simulink library "aerolib6dofsys"  (Simulink 5.0)
undefined symbols (not defined in the file or in its folder): e0_0, e1_0, e2_0, e3_0, eul_0, inertia, k_quat, mass_0, mass_e, mass_f
libraries: aerolibtransform2 x4, simulink x3, aerolibutil x1, aerolibbdyn x1
settings Model: Creator=sgage  LastModifiedBy=sgage  ExtModeAutoUpdateStatusClock=off  TargetHWChar=2  TargetHWWordLengths=8,16,32,32

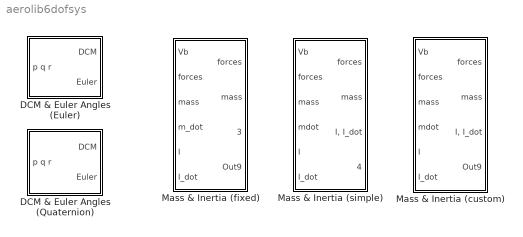
== system aerolib6dofsys ==
  DCM & Euler Angles (Euler) : Subsystem
      mask Type: DCM & Euler Angles (Euler)
  DCM & Euler Angles (Quaternion) : Subsystem
      mask Type: DCM & Euler Angles (Quaternion)
  Mass & Inertia (custom) : Subsystem
      mask Type: Mass & Inertia (custom)
  Mass & Inertia (fixed) : Subsystem
      mask Type: Mass & Inertia (fixed)
  Mass & Inertia (simple) : Subsystem
      mask Type: Mass & Inertia (simple)

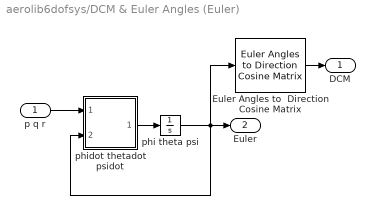
== system aerolib6dofsys/DCM & Euler Angles (Euler) ==
  "p q r " : Inport
  Euler Angles to  Direction Cosine Matrix : aerolibtransform2/Euler Angles to  Direction Cosine Matrix
  phi theta psi : Integrator  InitialCondition=eul_0
  phidot thetadot psidot : Subsystem
  DCM : Outport
  Euler : Outport  Port=2
  wires:
  Euler Angles to  Direction Cosine Matrix/1 -> DCM/1
  "p q r "/1 -> phidot thetadot psidot/1(p q r)
  phidot thetadot psidot/1(phidot thetadot psi) -> phi theta psi/1
  phi theta psi/1 -> Euler/1, phidot thetadot psidot/2(phi theta psi), Euler Angles to  Direction Cosine Matrix/1

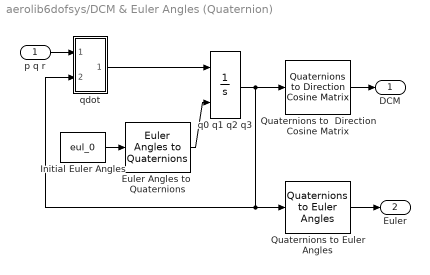
== system aerolib6dofsys/DCM & Euler Angles (Quaternion) ==
  p q r : Inport
  Euler Angles to  Quaternions : aerolibtransform2/Euler Angles to Quaternions
  Initial Euler Angles : Constant  Value=eul_0
  Quaternions to  Direction Cosine Matrix : aerolibtransform2/Quaternions to  Direction Cosine Matrix
  Quaternions to Euler Angles : aerolibtransform2/Quaternions to Euler Angles
  q0 q1 q2 q3 : Integrator  InitialConditionSource=external  InitialCondition=[e0_0 e1_0 e2_0 e3_0]
  qdot : Subsystem
  DCM : Outport
  Euler : Outport  Port=2
  wires:
  qdot/1(qdot) -> q0 q1 q2 q3/1
  q0 q1 q2 q3/1 -> qdot/2(q0 q1 q2 q3), Quaternions to Euler Angles/1, Quaternions to  Direction Cosine Matrix/1
  Euler Angles to  Quaternions/1 -> q0 q1 q2 q3/2
  Initial Euler Angles/1 -> Euler Angles to  Quaternions/1
  p q r/1 -> qdot/1(p q r)
  Quaternions to  Direction Cosine Matrix/1 -> DCM/1
  Quaternions to Euler Angles/1 -> Euler/1

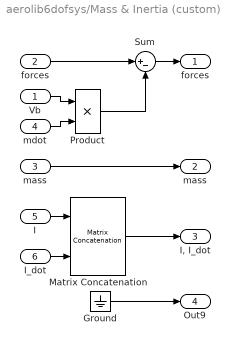
== system aerolib6dofsys/Mass & Inertia (custom) ==
  Vb : Inport
  forces : Inport  Port=2
  "mass " : Inport  Port=3
  mdot : Inport  Port=4
  I : Inport  Port=5
  I_dot : Inport  Port=6
  Ground : Ground
  Matrix Concatenation : simulink/Math Operations/Matrix Concatenation  numInports=2  catMethod=Vertical
  Product : Product  SaturateOnIntegerOverflow=on
  Sum : Sum  Inputs=|+-  SaturateOnIntegerOverflow=on
  "forces " : Outport
  mass : Outport  Port=2
  "I, I_dot " : Outport  Port=3
  Out9 : Outport  Port=4
  wires:
  Ground/1 -> Out9/1
  I/1 -> Matrix Concatenation/1
  "mass "/1 -> mass/1
  Matrix Concatenation/1 -> "I, I_dot "/1
  I_dot/1 -> Matrix Concatenation/2
  mdot/1 -> Product/2
  forces/1 -> Sum/1
  Vb/1 -> Product/1
  Sum/1 -> "forces "/1
  Product/1 -> Sum/2

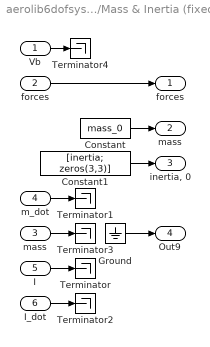
== system aerolib6dofsys/Mass & Inertia (fixed) ==
  Vb : Inport
  forces : Inport  Port=2
  "mass " : Inport  Port=3
  m_dot : Inport  Port=4  ShowAdditionalParam=on  DataType=double
  I : Inport  Port=5  ShowAdditionalParam=on  DataType=double
  I_dot : Inport  Port=6  ShowAdditionalParam=on  DataType=double
  Constant : Constant  Value=mass_0  ShowAdditionalParam=on
  Constant1 : Constant  Value=[inertia; zeros(3,3)]  ShowAdditionalParam=on
  Ground : Ground
  Terminator{,1..4} (5 alike) : Terminator
  "forces " : Outport
  mass : Outport  Port=2
  "inertia, 0" : Outport  Port=3
  Out9 : Outport  Port=4
  wires:
  Constant/1 -> mass/1
  Constant1/1 -> "inertia, 0"/1
  Ground/1 -> Out9/1
  I/1 -> Terminator/1
  m_dot/1 -> Terminator1/1
  I_dot/1 -> Terminator2/1
  "mass "/1 -> Terminator3/1
  forces/1 -> "forces "/1
  Vb/1 -> Terminator4/1

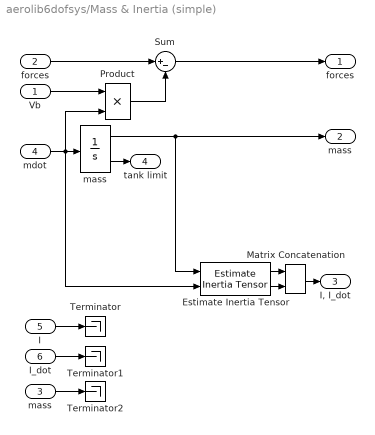
== system aerolib6dofsys/Mass & Inertia (simple) ==
  Vb : Inport
  forces : Inport  Port=2
  "mass " : Inport  Port=3
  mdot : Inport  Port=4
  I : Inport  Port=5  ShowAdditionalParam=on  DataType=double
  I_dot : Inport  Port=6  ShowAdditionalParam=on  DataType=double
  Estimate Inertia Tensor : aerolibbdyn/Estimate Inertia Tensor  fmass=mass_f  emass=mass_e  fI=inertia_f  eI=inertia_e
  Matrix Concatenation : simulink/Math Operations/Matrix Concatenation  numInports=2  catMethod=Vertical
  Product : Product  SaturateOnIntegerOverflow=on
  Sum : Sum  Inputs=|+-  SaturateOnIntegerOverflow=on
  Terminator : Terminator
  Terminator1 : Terminator
  Terminator2 : Terminator
  "mass  " : Integrator  InitialCondition=mass_0  LimitOutput=on  UpperSaturationLimit=mass_f  LowerSaturationLimit=mass_e  ShowSaturationPort=on
  "forces " : Outport
  mass : Outport  Port=2
  "I, I_dot" : Outport  Port=3
  tank limit : Outport  Port=4
  wires:
  "mass  "/2 -> tank limit/1
  "mass  "/1 -> mass/1, Estimate Inertia Tensor/1
  mdot/1 -> "mass  "/1, Product/2, Estimate Inertia Tensor/2
  Estimate Inertia Tensor/1 -> Matrix Concatenation/1
  I/1 -> Terminator/1
  Estimate Inertia Tensor/2 -> Matrix Concatenation/2
  Matrix Concatenation/1 -> "I, I_dot"/1
  I_dot/1 -> Terminator1/1
  "mass "/1 -> Terminator2/1
  forces/1 -> Sum/1
  Vb/1 -> Product/1
  Sum/1 -> "forces "/1
  Product/1 -> Sum/2

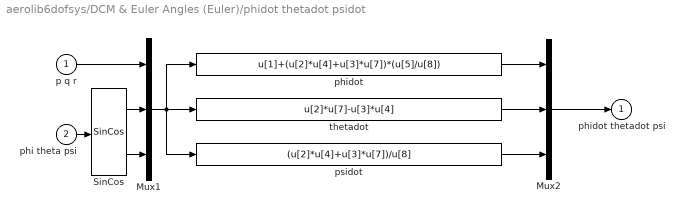
== system aerolib6dofsys/DCM & Euler Angles (Euler)/phidot thetadot psidot ==
  p q r : Inport
  phi theta psi : Inport  Port=2
  Mux1 : Mux  Inputs=[3 3 3]
  Mux2 : Mux  Inputs=3
  SinCos : aerolibutil/SinCos
  phidot : Fcn  Expr=u[1]+(u[2]*u[4]+u[3]*u[7])*(u[5]/u[8])
  psidot : Fcn  Expr=(u[2]*u[4]+u[3]*u[7])/u[8]
  thetadot : Fcn  Expr=u[2]*u[7]-u[3]*u[4]
  phidot thetadot psi : Outport  InitialOutput=0
  wires:
  SinCos/2 -> Mux1/3
  SinCos/1 -> Mux1/2
  Mux2/1 -> phidot thetadot psi/1
  phidot/1 -> Mux2/1
  thetadot/1 -> Mux2/2
  psidot/1 -> Mux2/3
  phi theta psi/1 -> SinCos/1
  p q r/1 -> Mux1/1
  Mux1/1 -> thetadot/1, phidot/1, psidot/1

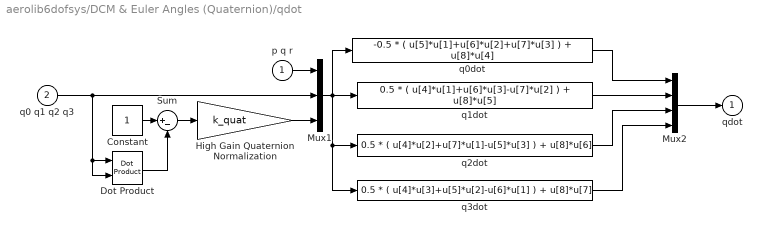
== system aerolib6dofsys/DCM & Euler Angles (Quaternion)/qdot ==
  p q r : Inport
  q0 q1 q2 q3 : Inport  Port=2
  Constant : Constant
  Dot Product : simulink/Math Operations/Dot Product  OutDataType=sfix(16)  OutScaling=2^-10  DoSatur=off
  High Gain Quaternion Normalization : Gain  Gain=k_quat  SaturateOnIntegerOverflow=on
  Mux1 : Mux  Inputs=[3 4 1]
  Mux2 : Mux
  Sum : Sum  Inputs=|+-  SaturateOnIntegerOverflow=on  InputSameDT=on
  q0dot : Fcn  Expr=-0.5 * ( u[5]*u[1]+u[6]*u[2]+u[7]*u[3] ) + u[8]*u[4]
  q1dot : Fcn  Expr=0.5 * ( u[4]*u[1]+u[6]*u[3]-u[7]*u[2] ) + u[8]*u[5]
  q2dot : Fcn  Expr=0.5 * ( u[4]*u[2]+u[7]*u[1]-u[5]*u[3] ) + u[8]*u[6]
  q3dot : Fcn  Expr=0.5 * ( u[4]*u[3]+u[5]*u[2]-u[6]*u[1] ) + u[8]*u[7]
  qdot : Outport  InitialOutput=0
  wires:
  q0 q1 q2 q3/1 -> Mux1/2, Dot Product/2, Dot Product/1
  q3dot/1 -> Mux2/4
  Mux1/1 -> q1dot/1, q0dot/1, q3dot/1, q2dot/1
  q2dot/1 -> Mux2/3
  q1dot/1 -> Mux2/2
  q0dot/1 -> Mux2/1
  Mux2/1 -> qdot/1
  Constant/1 -> Sum/1
  Sum/1 -> High Gain Quaternion Normalization/1
  High Gain Quaternion Normalization/1 -> Mux1/3
  Dot Product/1 -> Sum/2
  p q r/1 -> Mux1/1
